simulink model "exp03"  (R2018a)
settings: Solver=VariableStepAuto  StartTime=0.0  StopTime=10.0  RelTol=1e-3
settings Model: Creator=Administrator  LastModifiedBy=Administrator

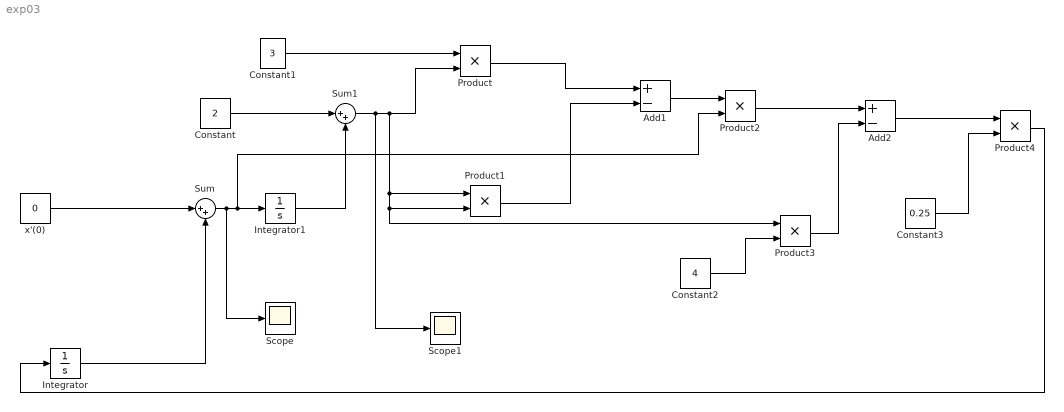
== system exp03 ==
  Add1 : Sum  Inputs=+-
  Add2 : Sum  Inputs=+-
  Constant : Constant  Value=2
  Constant1 : Constant  Value=3
  Constant2 : Constant  Value=4
  Constant3 : Constant  Value=0.25
  Integrator : Integrator
  Integrator1 : Integrator
  Product{,1..4} (5 alike) : Product
  Scope : Scope
  Scope1 : Scope
  Sum : Sum  Inputs=|++
  Sum1 : Sum  Inputs=|++
  x'(0) : Constant  Value=0
  wires:
  x'(0)/1 -> Sum/1
  Constant/1 -> Sum1/1
  Integrator/1 -> Sum/2
  Sum/1 -> Scope/1, Product2/2, Integrator1/1
  Integrator1/1 -> Sum1/2
  Constant1/1 -> Product/1
  Sum1/1 -> Scope1/1, Product3/1, Product1/2, Product1/1, Product/2
  Product/1 -> Add1/1
  Product1/1 -> Add1/2
  Add1/1 -> Product2/1
  Product2/1 -> Add2/1
  Constant2/1 -> Product3/2
  Product3/1 -> Add2/2
  Add2/1 -> Product4/1
  Constant3/1 -> Product4/2
  Product4/1 -> Integrator/1
